simulink model "FourOrderODE_Simulation"  (R2025b)
settings: Solver=ode45  StartTime=0.0  StopTime=100  MaxStep=0.1  RelTol=1e-3
settings Model: Creator=xhunl  LastModifiedBy=xhunl

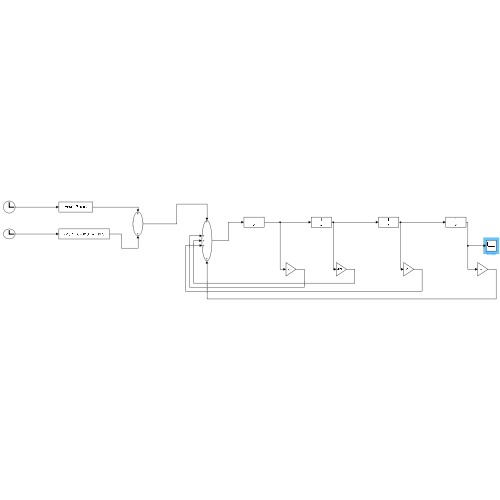
[thumbnail: Simulink's stored preview of the top-level diagram]
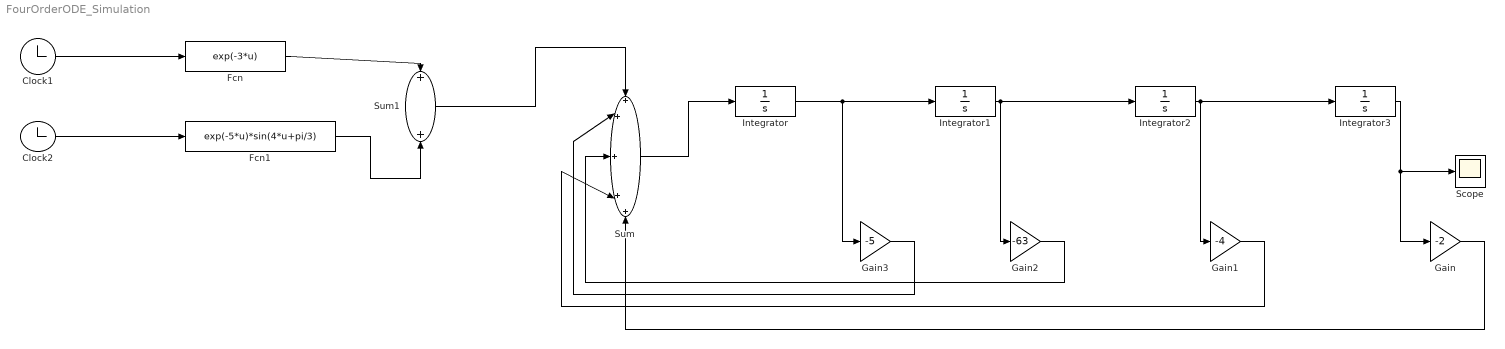
== system FourOrderODE_Simulation ==
  Clock1 : Clock
  Clock2 : Clock
  Fcn : Fcn  Expr=exp(-3*u)
  Fcn1 : Fcn  Expr=exp(-5*u)*sin(4*u+pi/3)
  Gain : Gain  Gain=-2
  Gain1 : Gain  Gain=-4
  Gain2 : Gain  Gain=-63
  Gain3 : Gain  Gain=-5
  Integrator : Integrator  InitialCondition=0.2
  Integrator1 : Integrator  InitialCondition=0.5
  Integrator2 : Integrator  InitialCondition=0.5
  Integrator3 : Integrator  InitialCondition=1
  Scope : Scope
      settings: ActiveDisplayYMinimum=-2.1942217653727427  ActiveDisplayYMaximum=3.3860577352171224
  Sum : Sum  Inputs=+++++
  Sum1 : Sum
  wires:
  Clock1/1 -> Fcn/1
  Clock2/1 -> Fcn1/1
  Fcn/1 -> Sum1/1
  Fcn1/1 -> Sum1/2
  Sum1/1 -> Sum/1
  Sum/1 -> Integrator/1
  Integrator/1 -> Integrator1/1, Gain3/1
  Integrator1/1 -> Integrator2/1, Gain2/1
  Integrator2/1 -> Integrator3/1, Gain1/1
  Gain3/1 -> Sum/2
  Gain2/1 -> Sum/3
  Gain1/1 -> Sum/4
  Integrator3/1 -> Scope/1, Gain/1
  Gain/1 -> Sum/5
